simulink model "ORR_Part2"  (R2024b)
settings: Solver=VariableStepAuto  StartTime=0.0  StopTime=10.0  RelTol=1e-3
values from neighbouring files (symbols this model uses):
  E_b_ECI_0 = [phi_b_eci_0; theta_b_eci_0; psi_b_eci_0]    [Final_4.m]    (also in Part3_Disturbance.m = C2EulerAngles(C_b_ECI_0); Part_2_TorqueFreeMotion_Orr.m = C2euler(C_b_eci_0); Part_3_Disturbance_ORR.m = C2euler(C_b_eci_0); Part_5_ORR.m = C2euler(C_b_eci_0))
  J = n.sat.I    [Part5_TorqueFreeMotion_SS.m]    (also in Part_2_TorqueFreeMotion_Orr.m = [812.0396         0         0; Part_5_ORR.m = [d.Ixx, d.Ixy, d.Ixz;         d.Ixy, d.Iyy, d.Iyz;         d)
  q_b_ECI_0 = q_b_ECI_0(:)    [Final_4.m]    (also in Part3_Disturbance.m = C2quat(C_b_ECI_0); Part_2_TorqueFreeMotion_Orr.m = C2quart(C_b_eci_0); Part_3_Disturbance_ORR.m = C2quat(C_b_eci_0); Part_5_ORR.m = C2quat(C_b_eci_0))
  T = T_c    [Final_3.m]    (also in ORR_part4_script.m; Part2_TorqueFreeMotion.m = [0;0;0]; Part2_TorqueFreeMotion_SS.m = [0;0;0]; Part5_TorqueFreeMotion_SS.m = [0;0;0])
  w_b_ECI_0 = w_b_ECI_0(:)    [Final_3.m]    (also in Final_4.m = [0.001; -0.001; 0.002]; ORR_part4_script.m = [0.001; -0.001; 0.002]; Part3_Disturbance.m = [0.001; -0.001; 0.002]; Part_2_TorqueFreeMotion_Orr.m = [0.001)
settings Model: Creator=haile  LastModifiedBy=haile

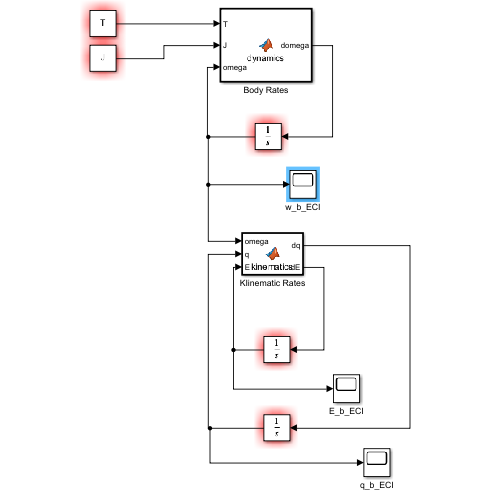
[thumbnail: Simulink's stored preview of the top-level diagram]
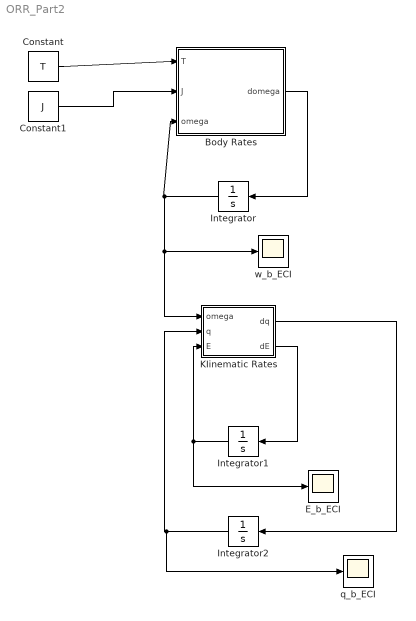
== system ORR_Part2 ==
  Body Rates : MATLAB Function  TreatAsAtomicUnit=on
  Constant : Constant  Value=T
  Constant1 : Constant  Value=J
  E_b_ECI : Scope
  Integrator : Integrator  InitialCondition=w_b_ECI_0
  Integrator1 : Integrator  InitialCondition=E_b_ECI_0
  Integrator2 : Integrator  InitialCondition=q_b_ECI_0
  KIinematic Rates : MATLAB Function  TreatAsAtomicUnit=on
  q_b_ECI : Scope
  w_b_ECI : Scope
  wires:
  Constant/1 -> Body Rates/1(T)
  Constant1/1 -> Body Rates/2(J)
  Body Rates/1(domega) -> Integrator/1
  Integrator/1 -> w_b_ECI/1, KIinematic Rates/1(omega), Body Rates/3(omega)
  KIinematic Rates/2(dE) -> Integrator1/1
  Integrator1/1 -> E_b_ECI/1, KIinematic Rates/3(E)
  KIinematic Rates/1(dq) -> Integrator2/1
  Integrator2/1 -> q_b_ECI/1, KIinematic Rates/2(q)

== matlab function ORR_Part2/KIinematic Rates ==
  data: omega input; dq output; q input; E input; dE output
function [dq, dE] = kinematics(omega, q, E)

    I = [1 0 0
        0 1 0
        0 0 1];

    omega = omega(:);
    E = E(:);
    q = q(:);
   
    theta_x = E(1);
    theta_y = E(2);
    %theta_z = e(3); not necessary in calculations

    epsilon = q(1:3);
    eta = q(4);

    C21 = [cos(theta_y) sin(theta_x) * sin(theta_y) cos(theta_x) * sin(theta_y)
      0 cos(theta_x) * cos(theta_y) -sin(theta_x) * cos(theta_y)
      0 sin(theta_x) cos(theta_x)];
    
    epsilon_dot = 0.5 * (eta * I * omega + cross(epsilon, omega));
    eta_dot = -0.5 * epsilon.' * omega;
    dq = [epsilon_dot; eta_dot];

    dE = (1 / cos(theta_y)) * C21 * omega;

end

== matlab function ORR_Part2/Body Rates ==
  data: T input; domega output; J input; omega input
function domega = dynamics(T, J, omega)

T = T(:);
omega = omega(:);

% step 1: use eulers equation to calculate angular velocity change
domega = inv(J) * (T - cross(omega, J*omega));


end
